simulink model "rov_kinematics_level0"  (R2024b)
settings: Solver=VariableStepAuto  StartTime=0.0  StopTime=10.0  RelTol=1e-3
settings Model: Creator=eirikvarnes  LastModifiedBy=eirikvarnes
settings DataIOCC: SaveFormat=Array  SaveTime=off  ReturnWorkspaceOutputs=off  OutputSaveName=eta

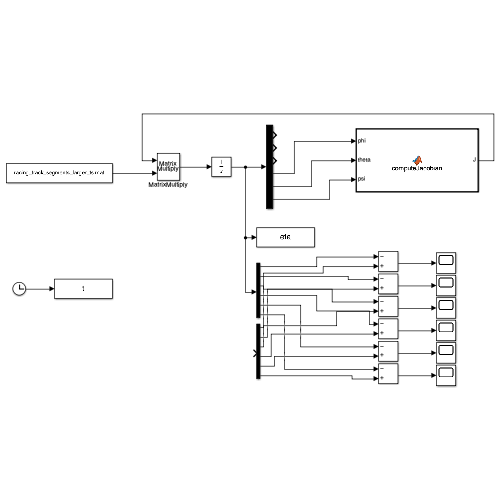
[thumbnail: Simulink's stored preview of the top-level diagram]
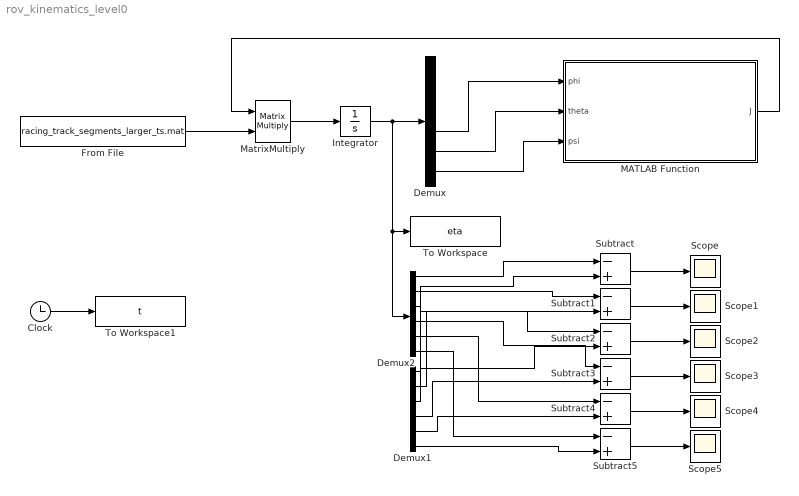
== system rov_kinematics_level0 ==
  Clock : Clock
  Demux : Demux  Outputs=6
  Demux1 : Demux  Outputs=6
  Demux2 : Demux  Outputs=6
  From File : FromFile  FileName=racing_track_segments_larger_ts.mat
  Integrator : Integrator
  MATLAB Function : MATLAB Function  TreatAsAtomicUnit=on
  MatrixMultiply : Product  Multiplication=Matrix(*)
  Scope{,1..5} (6 alike) : Scope
  Subtract{,1..5} (6 alike) : Sum  Inputs=-+
  To Workspace : ToWorkspace  VariableName=eta  SampleTime=-1
  To Workspace1 : ToWorkspace  VariableName=t  SampleTime=-1
  wires:
  MATLAB Function/1(J) -> MatrixMultiply/1
  Demux/4 -> MATLAB Function/1(phi)
  Demux/5 -> MATLAB Function/2(theta)
  Demux/6 -> MATLAB Function/3(psi)
  Integrator/1 -> Demux2/1, To Workspace/1, Demux/1
  MatrixMultiply/1 -> Integrator/1
  From File/1 -> MatrixMultiply/2
  Clock/1 -> To Workspace1/1
  Subtract/1 -> Scope/1
  Demux2/1 -> Subtract/1
  Demux1/1 -> Subtract/2
  Subtract1/1 -> Scope1/1
  Demux2/2 -> Subtract1/1
  Demux1/2 -> Subtract1/2
  Subtract2/1 -> Scope2/1
  Demux1/3 -> Subtract2/2
  Demux2/3 -> Subtract2/1
  Subtract3/1 -> Scope3/1
  Demux2/4 -> Subtract3/1
  Subtract4/1 -> Scope4/1
  Demux1/5 -> Subtract4/2
  Demux1/4 -> Subtract3/2
  Demux2/5 -> Subtract4/1
  Subtract5/1 -> Scope5/1
  Demux1/6 -> Subtract5/2
  Demux2/6 -> Subtract5/1

== matlab function rov_kinematics_level0/MATLAB Function ==
  data: phi input; J output; theta input; psi input
function J = computeJacobian(phi, theta, psi)

Rz = [cos(psi), -sin(psi), 0;
      sin(psi),  cos(psi), 0;
      0,         0,        1];
Ry = [cos(theta), 0, sin(theta);
      0,          1, 0;
     -sin(theta), 0, cos(theta)];
Rx = [1, 0,        0;
      0, cos(phi), -sin(phi);
      0, sin(phi),  cos(phi)];
R = Rz * Ry * Rx;

T = [1, sin(phi)*tan(theta), cos(phi)*tan(theta);
     0, cos(phi), -sin(phi);
     0, sin(phi)/cos(theta), cos(phi)/cos(theta)];

J = [R, zeros(3); zeros(3), T];
end
